simulink model "SimscapeModel3"  (R2023a)
settings: Solver=ode15s  StartTime=0.0  StopTime=inf  RelTol=1e-3
libraries: fl_lib x10, nesl_utility x4, arduinolib x3, simulink x1, arduinosensorlib x1
settings Model: Creator=moham  LastModifiedBy=moham
settings DataIOCC: ExternalInput=Adham.getElement(1)

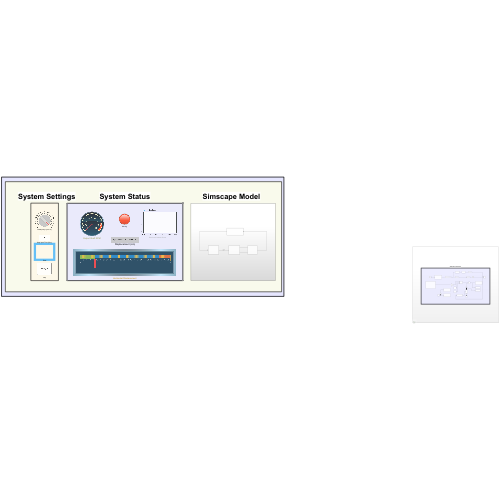
[thumbnail: Simulink's stored preview of the top-level diagram]
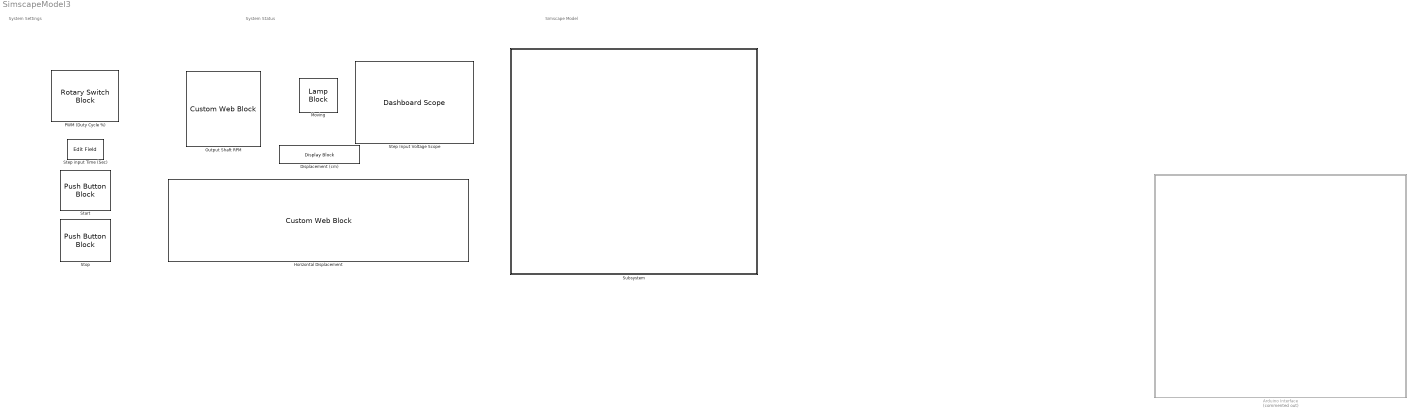
== system SimscapeModel3 ==
  note: System Settings
  note: System Status
  note: Simscape Model
  " Start" : PushButtonBlock  ButtonText=Start Step Input  IconAlignment=Center  OffValue=0.000000
  Arduino Interface : Subsystem  Commented=on
  Displacement (cm) : DisplayBlock  LabelPosition=Hide  Format=Custom  Transparency=1  FormatString=Displacement: %d cm
  Horizontal Displacement : CustomWebBlock  LabelPosition=Hide  ShowInitialText=on  Configuration="{\"components\":[{\"name\":\"LinearScaleComponent\",\"settings\":{\"bounds\":{\"max\":80,\"min\":0,\"tickInterval\":1},\"internalTickHeightScaleFactor\":0.5,\"labelColor\":[255,255,255],\"labelFont\":{\"font\":\"Arial\",\"fontSize\":12},\"labelOffset\":0.05,\"labelTransparency\":1,\"needleImage\":{\"size\":[21,75],\"src\":\"data:image\\/svg+xml;base64,PHN2ZyB4bWxucz0iaHR0cDovL3d3dy53My5vcmcvMjAwMC9zdmciIHhtbG5zOnhsaW5rPSJodHRwOi8vd3d3LnczLm9yZy8xOTk5L3hsaW5rIiB2aWV3Qm94PSIwIDAgMjEgNzUiPjxkZWZzPjxzdHlsZT4uY2xzLTF7ZmlsbDpub25lO30uY2xzLTJ7aXNvbGF0aW9uOmlzb2xhdGU7fS5jbHMtM3tjbGlwLXBhdGg6dXJsKCNjbGlwLXBhdGgpO30uY2xzLTR7b3BhY2l0eTowLjM7bWl4LWJsZW5kLW1vZGU6bXVsdGlwbHk7fS5jbHMtNXtmaWxsOiNlYjI2Mjk7fTwvc3R5bGU+PGNsaXBQYXRoIGlkPSJjbGlwLXBhdGgiIHRyYW5zZm9y ...(+1928 chars)\",\"srcOrientation\":\"Right\"},\"needleOffset\":[0.22707423580786026,-0.016333650491595308],\"needleSize\":{\"height\":0.4199677230046948,\"width\":0.06298064438807104},\"position\":[0.06964016965385142,0.01993022565320668,0.9712737529691211,0.5459023122178136],\"referencePoint\":\"auto\",\"scaleColors\":[{\"Color\":[0,114,189],\"Max\":70,\"Min\":0},{\"Color\":[217,83,25],\"Max\":80,\"Min\":70}],\"scaleColorsSize\":0.2,\"scaleDirection\":\"LR\",\"showLabels\":1,\"showMinorTicks\":0,\"showSpanLine\":1,\"showTicks\":1,\"tickColor\":[237,177,32],\"tickTransparency\":1,\"valueBarColor\":[119,172,48],\"valueBarOffset\":0,\"valueBarSize\":0.23,\"valueBarTransparency\":1}},{\"name\":\"BackgroundImageComponent\",\"settings\":{\"image\":{\"size\":[380,101],\"src\":\"data:image\\/svg+xml;base64,PHN2ZyBpZD0iZnJhbWUiIHhtbG5zPSJodHRwOi8vd3d3LnczLm9yZy8yMDAwL3N2ZyIgeG1sbnM6eGxpbms9Imh0dHA6Ly93d3cudzMub3JnLzE5OTkveGxpbmsiIHZpZXdCb3g9IjAgMCAzODAgMTAxIj48ZGVmcz48c3R5bGU+LmNscy0xe2ZpbGw6IzAwMmI0Mjt9LmNscy0ye2ZpbGw6IzQyNzA4Mjt9LmNscy0ze2ZpbGw6dXJsKCNyYWRpYWwtZ3JhZGllbnQpO308L3N0eWxlPjxyYWRpYWxHcmFkaWVudCBpZD0icmFkaWFsLWdyYWRpZW50IiBjeD0iMTkwIiBjeT0iNTAuNSIgcj0iMjY5LjIxIiBncmFkaWVudFVuaXRzPSJ1c2VyU3BhY2VPblVzZSI+PHN0b3Agb2Zmc2V0PSIwLjAxIiBzdG9wLWNvbG9yPSIjM2U0ZjU4Ii8+PHN0b3Agb2Zmc2V0PSIwLjA2IiBzdG9wLWNvbG9yPSIjNDQ1NzYxIi8+PHN0b3Agb2Zmc2V0PSIwLjE1IiBzdG9wLWNvbG9yPSIjNTU2YTc2Ii8+PHN0b3Agb2Zmc2V0PSIwLjI1IiBzdG9wLWNvbG9yPSIjNmQ4ODk1Ii8+PHN0b3Agb2Zmc2V0PSIwLjM4IiBzdG9wLWNvbG9yPSIjOGZiMmMzIi8+PHN0b3Agb2Zmc2V0PSIwLjUyIiBzdG9wLWNvbG9yPSIjYjZlNGZhIi8+PHN0b3Agb2Zmc2V0PSIxIiBzdG9wLWNvbG9yPSIjMTU0NjU3Ii8+PC9yYWRpYWxHcmFkaWVudD48L2RlZnM+PGcgaWQ9IkxheWVyXzIiIGRhdGEtbmFtZT0iTGF5ZXIgMiI+PGcgaWQ9IkxheWVyXzEtMiIgZGF0YS1uYW1lPSJMYXllciAxLTIiPjxyZWN0IGlkPSJyZWN0MTAzNiIgY2xhc3M9ImNscy0xIiB4PSIxMSIgeT0iMTEiIHdpZHRoPSIzNTgiIGhlaWdodD0iNzkiLz48cGF0aCBpZD0icGF0aDEwMzgiIGNsYXNzPSJjbHMtMiIgZD0iTTgsOFY5M0gzNzJWOFpNMzY5LDkwSDExVjExSDM2OVoiLz48cGF0aCBpZD0icGF0aDEwNDAiIGNsYXNzPSJjbHMtMyIgZD0iTTAsMFYxMDFIMzgwVjBaTTM3Miw5M0g4VjhIMzcyWiIvPjwvZz48L2c+PC9zdmc+\",\"srcOrientation\":\"Right\"},\"position\":[0,0,1,1],\"scaleMode\":\"0\"}},{\"name\":\"ForegroundImageComponent\",\"settings\":{\"angle\":0,\"image\":{\"size\":[457,124],\"src\":\"default\",\"srcOrientation\":null},\"isForeground\":1,\"position\":[0,0,1,1],\"scaleMode\":\"0\"}}],\"settings\":{\"BindingType\":\"signal\",\"backgroundColor\":[0,0,0,\"1\"],\"backgroundOffset\":0,\"backgroundOpacity\":1,\"fixedAspectRatio\":\"on\",\"orientation\":\"horizontal\",\"showBackgroundColor\":false,\"value\":0,\"version\":\"R2023a\"},\"type\":\"LinearGauge\"}"
  Moving : LampBlock  LabelPosition=Hide
  Output Shaft RPM : CustomWebBlock  LabelPosition=Hide  ShowInitialText=on  Configuration="{\"components\":[{\"name\":\"CircularScaleComponent\",\"settings\":{\"bounds\":{\"max\":80,\"min\":0,\"tickInterval\":\"auto\"},\"direction\":\"cw\",\"flipLimits\":0,\"innerRadius\":0.75,\"internalTickHeightScaleFactor\":1,\"labelColor\":[255,255,200],\"labelFont\":{\"font\":\"Arial\",\"fontSize\":12},\"labelRadius\":0.528,\"labelTransparency\":1,\"minorTickHeightScaleFactor\":0.2,\"needleImage\":{\"size\":[200,50],\"src\":\"data:image\\/svg+xml;base64,PD94bWwgdmVyc2lvbj0iMS4wIiBlbmNvZGluZz0idXRmLTgiPz4KPCEtLSBHZW5lcmF0b3I6IEFkb2JlIElsbHVzdHJhdG9yIDI0LjEuMiwgU1ZHIEV4cG9ydCBQbHVnLUluIC4gU1ZHIFZlcnNpb246IDYuMDAgQnVpbGQgMCkgIC0tPgo8c3ZnIHZlcnNpb249IjEuMSIgaWQ9IkxheWVyXzEiIHhtbG5zPSJodHRwOi8vd3d3LnczLm9yZy8yMDAwL3N2ZyIgeG1sbnM6eGxpbms9Imh0dHA6Ly93d3cudzMub3JnLzE5OTkveGxpbmsiIHg9IjBweCIgeT0iMHB4IgoJIHZpZXdCb3g9IjAgMCAyMDAgNTAiIHN0eWxlPSJlbmFibGUtYmFja2dyb3VuZDpuZXcgMCAwIDIwMCA1MDsiIHhtbDpzcGFjZT0icHJlc2VydmUiPgo8c3R5bGUgdHlwZT0idGV4dC9jc3MiPgoJLnN0MHtmaWxsOiNFQzIxMjc7fQo8L3N0eWxlPgo8cGF0aCBjbGFzcz0ic3QwIiBkPSJNMTYyLjgsMTMuN0MxNjksNC40LDE4MS43LDEuOSwxOTEsOC4xczExLjgsMTguOSw1LjYsMjguMnMtMTguOSwxMS44LTI4LjIsNS42bDAsMAoJQzE1OS4xLDM1LjYsMTU2LjYsMjMsMTYyLjgsMTMuN0wxNjIuOCwxMy43eiBNMTY1LjgsMTUuOGMtNS4xLDcuNi0zLjEsMTcuOSw0LjYsMjNjNy42LDUuMSwxNy45LDMuMSwyMy00LjYKCWM1LjEtNy42LDMuMS0xNy45LTQuNi0yM2wwLDBDMTgxLjIsNi4yLDE3MC45LDguMiwxNjUuOCwxNS44eiIvPgo8cGF0aCBjbGFzcz0ic3QwIiBkPSJNMC40LDI1Ljl2LTMuM2wxNTktMi41Yy0wLjcsMi42LTAuNyw1LjIsMCw3LjhMMC40LDI1Ljl6Ii8+CjxjaXJjbGUgY2xhc3M9InN0MCIgY3g9IjE3OS42IiBjeT0iMjQiIHI9IjAuNyIvPgo8L3N2Zz4K\"},\"needleOffset\":[0.18464878250906522,0],\"needleOrientation\":-45,\"needleRotation\":180,\"needleSize\":{\"height\":0.11741692305346914,\"width\":0.46108337545091255},\"outerRadius\":0.9,\"position\":[0.05,0.05,0.9,0.9],\"referencePoint\":\"auto\",\"scaleAngle\":270,\"scaleAngleOffset\":135,\"scaleColors\":[{\"Color\":[254,51,10],\"Max\":80,\"Min\":65}],\"scaleColorsSize\":0.2,\"scaleDirection\":\"CW\",\"scalePosition\":[0,0,1,1],\"showLabels\":1,\"showMinorTicks\":1,\"showSpanLine\":1,\"showTicks\":1,\"tickColor\":[252,252,197],\"tickTransparency\":1,\"valueBarColor\":[0,114,189],\"valueBarPosition\":[0,0,1,1],\"valueBarSize\":0.2,\"valueBarTransparency\":1}},{\"name\":\"BackgroundImageComponent\",\"settings\":{\"image\":{\"size\":[500,500],\"src\":\"data:image\\/svg+xml;base64,PD94bWwgdmVyc2lvbj0iMS4wIiBlbmNvZGluZz0iVVRGLTgiIHN0YW5kYWxvbmU9Im5vIj8+CjxzdmcKICAgeG1sbnM6ZGM9Imh0dHA6Ly9wdXJsLm9yZy9kYy9lbGVtZW50cy8xLjEvIgogICB4bWxuczpjYz0iaHR0cDovL2NyZWF0aXZlY29tbW9ucy5vcmcvbnMjIgogICB4bWxuczpyZGY9Imh0dHA6Ly93d3cudzMub3JnLzE5OTkvMDIvMjItcmRmLXN5bnRheC1ucyMiCiAgIHhtbG5zOnN2Zz0iaHR0cDovL3d3dy53My5vcmcvMjAwMC9zdmciCiAgIHhtbG5zPSJodHRwOi8vd3d3LnczLm9yZy8yMDAwL3N2ZyIKICAgeG1sbnM6 ...(+9964 chars)\"},\"position\":[0,0,1,1],\"scaleMode\":\"0\"}},{\"name\":\"ForegroundImageComponent\",\"settings\":{\"image\":{\"size\":[0,0],\"src\":\"default\",\"srcOrientation\":[]},\"isForeground\":1,\"position\":[0,0,1,1],\"scaleMode\":\"0\"}}],\"settings\":{\"BindingType\":\"signal\",\"aspectRatio\":1.032258064516129,\"backgroundColor\":[0,0,0,\"1\"],\"backgroundOffset\":1,\"backgroundOpacity\":1,\"direction\":\"cw\",\"fixedAspectRatio\":\"on\",\"flipLimits\":0,\"orientation\":\"horizontal\",\"showBackgroundColor\":false,\"value\":0,\"version\":\"R2023a\"},\"type\":\"CircularGauge\"}"
  PWM (Duty Cycle %) : RotarySwitchBlock  LabelPosition=Hide
      settings: Values={{'Off', '5', '10', '15', '20', '25', '30', '35', '40', '45', '50', '55', '60', '65', '70', '75', '80', '85', '90', '95', '100'}, [0 0.25 0.5 0.75 1 1.25 1.5 1.75 2 2.25 2.5 2.75 3 3.25 3.5 3.75 4 4.25 4.5 4.75 5]}
  Step Input Voltage Scope : DashboardScope  Ymin=0  Ymax=5.5
  Step input Time (Sec) : EditField  LabelPosition=Hide  ShowInitialText=on  Alignment=Center
  Stop : PushButtonBlock  ButtonText=Emergency Stop  OnValue=2  ButtonType=Latch  OffValue=0.000000
  Subsystem : Subsystem

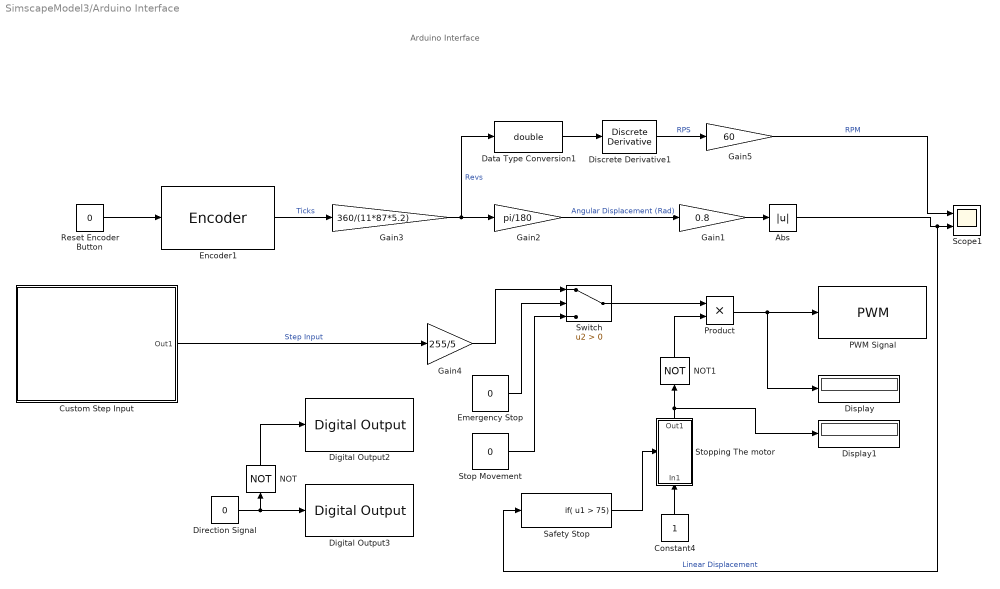
== system SimscapeModel3/Arduino Interface ==
  note: Arduino Interface
  Abs : Abs  SaturateOnIntegerOverflow=off
  Constant4 : Constant
  "Custom Step Input " : Subsystem
  Data Type Conversion1 : DataTypeConversion  OutDataTypeStr=double  SaturateOnIntegerOverflow=off  RndMeth=Floor
  Digital Output2 : arduinolib/Digital Output  pinNumber=8  Direction=output  blockPlatform=arduino
  Digital Output3 : arduinolib/Digital Output  pinNumber=7  Direction=output  blockPlatform=arduino
  Direction Signal : Constant  Value=0
  Discrete Derivative1 : simulink/Discrete/Discrete Derivative  gainval=1.0  ICPrevScaledInput=0.0  OutMin=[]  OutMax=[]  OutDataType=fixdt(1, 16)  OutScaling=2^-10  DoSatur=off
  Display : Display
  Display1 : Display
  Emergency Stop : Constant  Value=0
  Encoder1 : arduinosensorlib/Encoder  InputA=2  InputB=3  Mode=Reset by external signal  SampleTime=-1
  Gain1 : Gain  Gain=0.8  ParamDataTypeStr=double  OutDataTypeStr=double
  Gain2 : Gain  Gain=pi/180  ParamDataTypeStr=double  OutDataTypeStr=double
  Gain3 : Gain  Gain=360/(11*87*5.2)  ParamDataTypeStr=double  OutDataTypeStr=double
  Gain4 : Gain  Gain=255/5
  Gain5 : Gain  Gain=60  ParamDataTypeStr=double  OutDataTypeStr=double
  NOT : Logic  Operator=NOT  IconShape=distinctive  AllPortsSameDT=off  OutDataTypeStr=boolean
  NOT1 : Logic  Operator=NOT  IconShape=distinctive  AllPortsSameDT=off  OutDataTypeStr=boolean
  PWM Signal : arduinolib/PWM  pinNumber=5  frequencyType=Default  desiredFrequency=490.2  achievableFrequency=490.2
  Product : Product
  Reset Encoder Button : Constant  Value=0
  Safety Stop : If  IfExpression=u1 > 75  ShowElse=off
  Scope1 : Scope  NumInputPorts=2
  Stop Movement : Constant  Value=0
  Stopping The motor : Subsystem  TreatAsAtomicUnit=on
  Switch : Switch  Criteria=u2 > Threshold  SaturateOnIntegerOverflow=off  InputSameDT=off
  wires:
  NOT1/1 -> Product/2
  Product/1 -> Display/1, PWM Signal/1
  Gain4/1 -> Switch/1
  Constant4/1 -> Stopping The motor/1(In1)
  Encoder1/1 -> Gain3/1  "Ticks"
  Gain2/1 -> Gain1/1  "Angular Displacement (Rad)"
  Gain3/1 -> Gain2/1, Data Type Conversion1/1  "Revs"
  Safety Stop/1 -> Stopping The motor/Action
  Abs/1 -> Safety Stop/1, Scope1/2  "Linear Displacement"
  Stopping The motor/1(Out1) -> Display1/1, NOT1/1
  Reset Encoder Button/1 -> Encoder1/1
  Gain1/1 -> Abs/1
  "Custom Step Input "/1(Out1) -> Gain4/1  "Step Input"
  Switch/1 -> Product/1
  Stop Movement/1 -> Switch/3
  Emergency Stop/1 -> Switch/2
  Data Type Conversion1/1 -> Discrete Derivative1/1
  Discrete Derivative1/1 -> Gain5/1  "RPS"
  Gain5/1 -> Scope1/1  "RPM"
  Direction Signal/1 -> NOT/1, Digital Output3/1
  NOT/1 -> Digital Output2/1

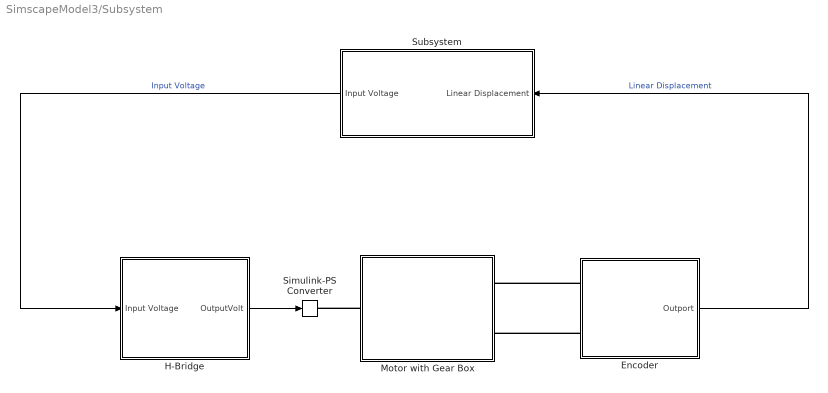
== system SimscapeModel3/Subsystem ==
  Encoder : Subsystem
      mask Display: image('$imagefile'); % Use "Edit Image" on toolstrip to change.
  H-Bridge : Subsystem
      mask Display: image('$imagefile'); % Use "Edit Image" on toolstrip to change.
  Motor with Gear Box : Subsystem
      mask Display: image('$imagefile'); % Use "Edit Image" on toolstrip to change.
  Simulink-PS Converter : nesl_utility/Simulink-PS Converter  PhysicalDomain=network_engine_domain  SubClassName=ps_input  LeftPortType=input  RightPortType=output  PseudoPeriodic=off  Frequencies=[]  NoiseDistribution=none  NoiseParameters=[]  Unit=1  AffineConversion=off  FilteringAndDerivatives=provide  SimscapeFilterOrder=1  InputFilterTimeConstant=0.001  UdotUserProvided=0
  Subsystem : Subsystem
  wires:
  Encoder/1(Outport) -> Subsystem/1(Linear Displacement)  "Linear Displacement"
  H-Bridge/1(OutputVolt) -> Simulink-PS Converter/1
  Subsystem/1(Input Voltage) -> H-Bridge/1(Input Voltage)  "Input Voltage"
  connections:
  Motor with Gear Box/RConn1 -- Simulink-PS Converter/RConn1
  Encoder/LConn1 -- Motor with Gear Box/LConn1
  Encoder/LConn2 -- Motor with Gear Box/LConn2

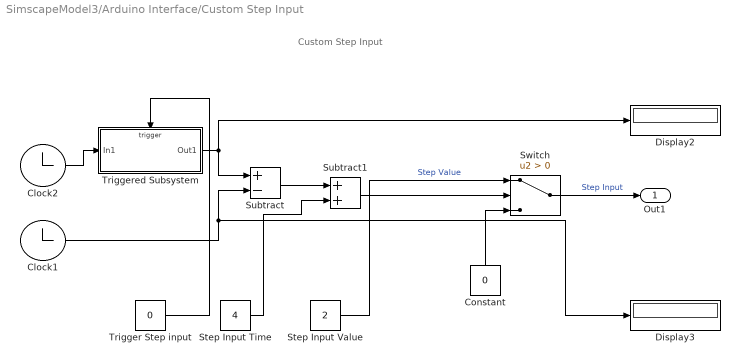
== system SimscapeModel3/Arduino Interface/Custom Step Input  ==
  note: Custom Step Input
  Clock1 : Clock
  Clock2 : Clock
  Constant : Constant  Value=0
  Display2 : Display
  Display3 : Display
  Step Input Time : Constant  Value=4
  Step Input Value : Constant  Value=2
  Subtract : Sum  Inputs=+-  OutMin=[400]
  Subtract1 : Sum  OutMin=[400]
  Switch : Switch  Criteria=u2 > Threshold  SaturateOnIntegerOverflow=off  InputSameDT=off
  Trigger Step input : Constant  Value=0
  Triggered Subsystem : Subsystem  TreatAsAtomicUnit=on
  Out1 : Outport
  wires:
  Step Input Value/1 -> Switch/1  "Step Value"
  Clock1/1 -> Subtract/2, Display3/1
  Subtract/1 -> Subtract1/1
  Triggered Subsystem/1(Out1) -> Subtract/1, Display2/1
  Trigger Step input/1 -> Triggered Subsystem/Trigger
  Constant/1 -> Switch/3
  Switch/1 -> Out1/1  "Step Input"
  Clock2/1 -> Triggered Subsystem/1(In1)
  Step Input Time/1 -> Subtract1/2
  Subtract1/1 -> Switch/2

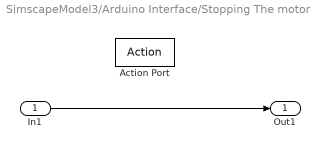
== system SimscapeModel3/Arduino Interface/Stopping The motor ==
  In1 : Inport
  Action Port : ActionPort
  Out1 : Outport
  wires:
  In1/1 -> Out1/1

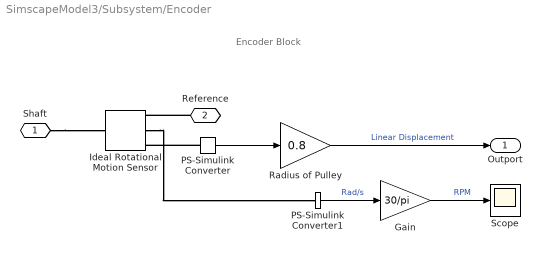
== system SimscapeModel3/Subsystem/Encoder ==
  note: Encoder Block
  Gain : Gain  Gain=30/pi
  Ideal Rotational Motion Sensor : fl_lib/Mechanical/Mechanical Sensors/Ideal Rotational Motion Sensor  reference=foundation.enum.MeasurementReference.difference  acceleration_port=false  velocity_port=true  position_port=true  wrap_angle=false  offset=0 rad
  PS-Simulink Converter : nesl_utility/PS-Simulink Converter  PhysicalDomain=network_engine_domain  SubClassName=ps_output  LeftPortType=input  RightPortType=output  PseudoPeriodic=off  Frequencies=[]  VectorFormat=inherit  Unit=inherit  AffineConversion=off
  PS-Simulink Converter1 : nesl_utility/PS-Simulink Converter  PhysicalDomain=network_engine_domain  SubClassName=ps_output  LeftPortType=input  RightPortType=output  PseudoPeriodic=off  Frequencies=[]  VectorFormat=inherit  Unit=inherit  AffineConversion=off
  Radius of Pulley : Gain  Gain=0.8
  Scope : Scope
  Shaft : PMIOPort  Side=Left
  Reference : PMIOPort  Port=2  Side=Left
  Outport : Outport
  wires:
  PS-Simulink Converter/1 -> Radius of Pulley/1
  Radius of Pulley/1 -> Outport/1  "Linear Displacement"
  PS-Simulink Converter1/1 -> Gain/1  "Rad/s"
  Gain/1 -> Scope/1  "RPM"
  connections:
  PS-Simulink Converter/LConn1 -- Ideal Rotational Motion Sensor/RConn3
  Shaft/RConn1 -- Ideal Rotational Motion Sensor/LConn1
  Reference/RConn1 -- Ideal Rotational Motion Sensor/RConn1
  Ideal Rotational Motion Sensor/RConn2 -- PS-Simulink Converter1/LConn1

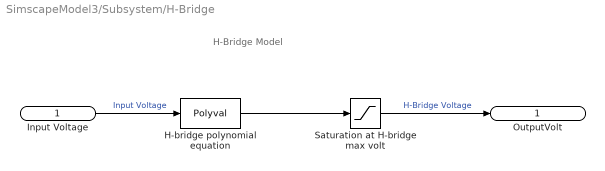
== system SimscapeModel3/Subsystem/H-Bridge ==
  note: H-Bridge Model
  Input Voltage : Inport
  H-bridge polynomial equation : Polyval  Coefs=[0.2132 -2.4754 10.0868 -4.4846]
  Saturation at H-bridge max volt : Saturate  UpperLimit=10.78  LowerLimit=0
  OutputVolt : Outport
  wires:
  Saturation at H-bridge max volt/1 -> OutputVolt/1  "H-Bridge Voltage"
  Input Voltage/1 -> H-bridge polynomial equation/1  "Input Voltage"
  H-bridge polynomial equation/1 -> Saturation at H-bridge max volt/1

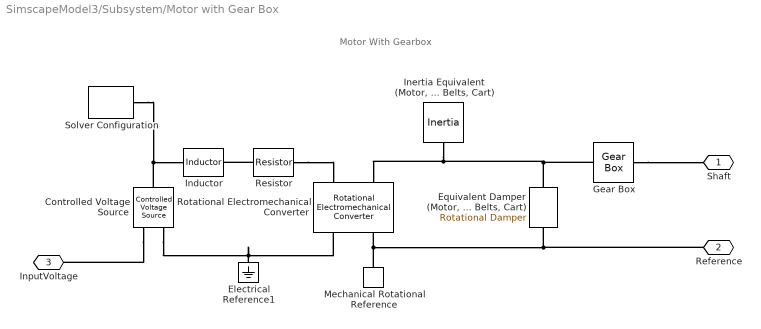
== system SimscapeModel3/Subsystem/Motor with Gear Box ==
  note: Motor With Gearbox
  Controlled Voltage Source : fl_lib/Electrical/Electrical Sources/Controlled Voltage Source
  Electrical Reference1 : fl_lib/Electrical/Electrical Elements/Electrical Reference
  "Equivalent Damper (Motor, Pulleys, Belts, Cart)" : fl_lib/Mechanical/Rotational Elements/Rotational Damper  D=1.1648e-05 N*m*s/rad  w_specify=off  w_priority=None  w=0 rad/s  w_nominal_specify=off  w_nominal_unit=rad/s  w_nominal_value=1  t_specify=off  t_priority=None  t=0 N*m  t_nominal_specify=off  t_nominal_unit=N*m  t_nominal_value=1
  Gear Box : fl_lib/Mechanical/Mechanisms/Gear Box  ratio=87  t_in_specify=off  t_in_priority=None  t_in=0 N*m  t_in_nominal_specify=off  t_in_nominal_unit=N*m  t_in_nominal_value=1  t_out_specify=off  t_out_priority=None  t_out=0 N*m  t_out_nominal_specify=off  t_out_nominal_unit=N*m  t_out_nominal_value=1
  Inductor : fl_lib/Electrical/Electrical Elements/Inductor  l=0.0097668 mH  r=0 Ohm  g=0 1/Ohm  i_specify=off  i_priority=None  i=0 A  i_nominal_specify=off  i_nominal_unit=A  i_nominal_value=1  v_specify=off  v_priority=None  v=0 V  v_nominal_specify=off  v_nominal_unit=V  v_nominal_value=1  i_L_specify=off  i_L_priority=High  i_L=0 A  i_L_nominal_specify=off  i_L_nominal_unit=A  i_L_nominal_value=1
  "Inertia Equivalent (Motor, Pulleys, Belts, Cart)" : fl_lib/Mechanical/Rotational Elements/Inertia  inertia=8.7499e-06 kg*m^2  num_ports=foundation.enum.numPorts2.one  w_specify=off  w_priority=High  w=0 rad/s  w_nominal_specify=off  w_nominal_unit=rad/s  w_nominal_value=1  t_specify=off  t_priority=None  t=0 N*m  t_nominal_specify=off  t_nominal_unit=N*m  t_nominal_value=1
  Mechanical Rotational Reference : fl_lib/Mechanical/Rotational Elements/Mechanical Rotational Reference
  Resistor : fl_lib/Electrical/Electrical Elements/Resistor  R=6 Ohm  i_specify=off  i_priority=None  i=0 A  i_nominal_specify=off  i_nominal_unit=A  i_nominal_value=1  v_specify=off  v_priority=None  v=0 V  v_nominal_specify=off  v_nominal_unit=V  v_nominal_value=1
  Rotational Electromechanical Converter : fl_lib/Electrical/Electrical Elements/Rotational Electromechanical Converter  K=0.018772 V*s/rad  i_specify=off  i_priority=None  i=0 A  i_nominal_specify=off  i_nominal_unit=A  i_nominal_value=1  v_specify=on  v_priority=None  v=0 V  v_nominal_specify=off  v_nominal_unit=V  v_nominal_value=1  t_specify=off  t_priority=None  t=0 N*m  t_nominal_specify=off  t_nominal_unit=N*m  t_nominal_value=1  w_specify=off  w_priority=None  w=0 rad/s  w_nominal_specify=off  w_nominal_unit=rad/s  w_nominal_value=1
  Solver Configuration : nesl_utility/Solver Configuration  PhysicalDomain=network_engine_domain  SubClassName=solver  LeftPortType=input  RightPortType=generic  Tones=[]  Harmonics=[]  SimulateNoise=off  Profile=off  UseLocalSampling=off  EnableSwitchedLinearOptims=on  FrequencyDomain=off  UseCCode=off  RelTol=0.001  AbsTol=0.001  MinStep=1e-09  ToWorkspace=off  RevertToSquareIcSolve=off  NumHomotopyIterations=100  PhasorMode=off  PhasorModeNumHarmonics=1  ConsistencySolver=NEWTON_XTOL_AFTER_FTOL  IndexReductionMethod=DerivativeReplacement  DoDC=off  ResidualTolerance=1e-09  ConsistencyTolSource=GLOBAL  ConsistencyAbsTol=0.001  ConsistencyRelTol=0.001  ConsistencyTolFactor=0.001  UseLocalSolver=off  LocalSolverChoice=NE_BACKWARD_EULER_ADVANCER  ResolveIndetEquations=on  FunctionEvalNumThread=1  LocalSolverSampleTime=0.001  DoFixedCost=off  MaxNonlinIter=3  MaxModeIter=2  ComputeImpulses=off  ImpulseIterations=2  LinearAlgebra=auto  LinearAlgebraNumThread=0  EquationFormulation=NE_TIME_EF  DelaysMemoryBudget=1024  AutomaticFiltering=on  FilteringTimeConstant=0.001  PartitionStorageMethod=AS_NEEDED  PartitionMemoryBudget=1024  PartitionMethod=ROBUST
  Shaft : PMIOPort  Side=Left
  Reference : PMIOPort  Port=2  Side=Left
  InputVoltage : PMIOPort  Port=3  Side=Right
  connections:
  Gear Box/RConn1 -- Shaft/RConn1
  Electrical Reference1/LConn1 -- Controlled Voltage Source/RConn2 -- Rotational Electromechanical Converter/RConn1
  Resistor/LConn1 -- Inductor/RConn1
  Solver Configuration/RConn1 -- Controlled Voltage Source/LConn1 -- Inductor/LConn1
  "Equivalent Damper (Motor, Pulleys, Belts, Cart)"/LConn1 -- "Inertia Equivalent (Motor, Pulleys, Belts, Cart)"/LConn1 -- Rotational Electromechanical Converter/LConn2 -- Gear Box/LConn1
  Controlled Voltage Source/RConn1 -- InputVoltage/RConn1
  Resistor/RConn1 -- Rotational Electromechanical Converter/LConn1
  Mechanical Rotational Reference/LConn1 -- Rotational Electromechanical Converter/RConn2 -- Reference/RConn1 -- "Equivalent Damper (Motor, Pulleys, Belts, Cart)"/RConn1

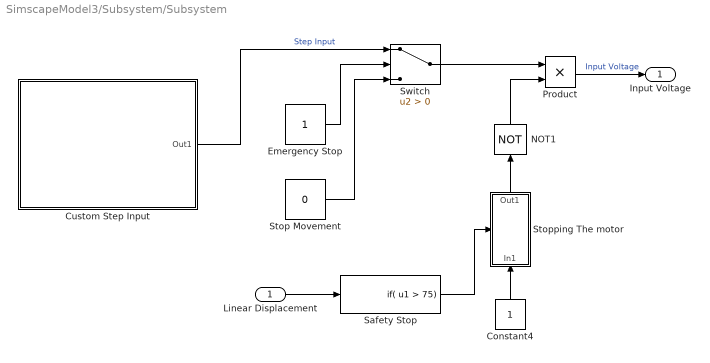
== system SimscapeModel3/Subsystem/Subsystem ==
  Linear Displacement : Inport
  Constant4 : Constant
  "Custom Step Input " : Subsystem
  Emergency Stop : Constant
  NOT1 : Logic  Operator=NOT  IconShape=distinctive  AllPortsSameDT=off  OutDataTypeStr=boolean
  Product : Product
  Safety Stop : If  IfExpression=u1 > 75  ShowElse=off
  Stop Movement : Constant  Value=0
  Stopping The motor : Subsystem  TreatAsAtomicUnit=on
  Switch : Switch  Criteria=u2 > Threshold  SaturateOnIntegerOverflow=off  InputSameDT=off
  Input Voltage : Outport
  wires:
  Stopping The motor/1(Out1) -> NOT1/1
  Safety Stop/1 -> Stopping The motor/Action
  Switch/1 -> Product/1
  Constant4/1 -> Stopping The motor/1(In1)
  Emergency Stop/1 -> Switch/2
  Stop Movement/1 -> Switch/3
  Linear Displacement/1 -> Safety Stop/1
  NOT1/1 -> Product/2
  Product/1 -> Input Voltage/1  "Input Voltage"
  "Custom Step Input "/1(Out1) -> Switch/1  "Step Input"

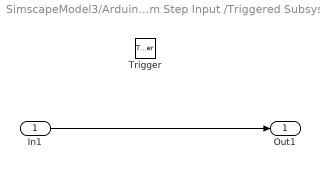
== system SimscapeModel3/Arduino Interface/Custom Step Input /Triggered Subsystem ==
  In1 : Inport
  Trigger : TriggerPort  VariantControl=(inherit)
  Out1 : Outport
  wires:
  In1/1 -> Out1/1

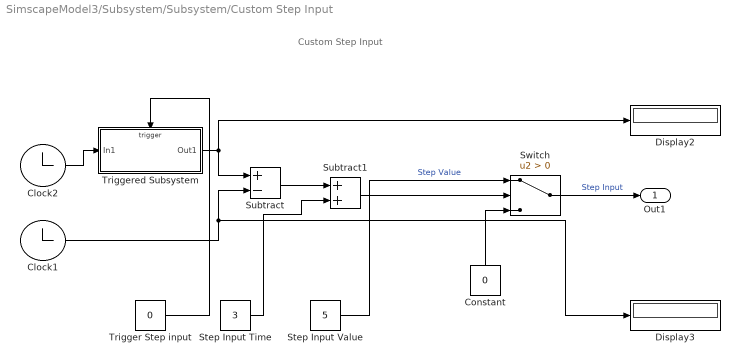
== system SimscapeModel3/Subsystem/Subsystem/Custom Step Input  ==
  note: Custom Step Input
  Clock1 : Clock
  Clock2 : Clock
  Constant : Constant  Value=0
  Display2 : Display
  Display3 : Display
  Step Input Time : Constant  Value=3
  Step Input Value : Constant  Value=5
  Subtract : Sum  Inputs=+-  OutMin=[400]
  Subtract1 : Sum  OutMin=[400]
  Switch : Switch  Criteria=u2 > Threshold  SaturateOnIntegerOverflow=off  InputSameDT=off
  Trigger Step input : Constant  Value=0
  Triggered Subsystem : Subsystem  TreatAsAtomicUnit=on
  Out1 : Outport
  wires:
  Step Input Value/1 -> Switch/1  "Step Value"
  Clock1/1 -> Subtract/2, Display3/1
  Subtract/1 -> Subtract1/1
  Triggered Subsystem/1(Out1) -> Subtract/1, Display2/1
  Trigger Step input/1 -> Triggered Subsystem/Trigger
  Constant/1 -> Switch/3
  Switch/1 -> Out1/1  "Step Input"
  Clock2/1 -> Triggered Subsystem/1(In1)
  Step Input Time/1 -> Subtract1/2
  Subtract1/1 -> Switch/2

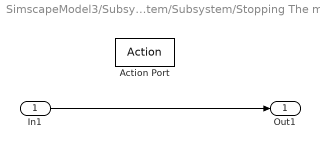
== system SimscapeModel3/Subsystem/Subsystem/Stopping The motor ==
  In1 : Inport
  Action Port : ActionPort  ActionPortLabel=if( u1 > 75)
  Out1 : Outport
  wires:
  In1/1 -> Out1/1

== system SimscapeModel3/Subsystem/Subsystem/Custom Step Input /Triggered Subsystem ==
  In1 : Inport
  Trigger : TriggerPort  VariantControl=(inherit)
  Out1 : Outport
  wires:
  In1/1 -> Out1/1
